simulink model "smc_controller"  (R2021a)
settings: Solver=VariableStepAuto  StartTime=0.01  StopTime=10  RelTol=1e-3
settings Model: Creator=Admin  LastModifiedBy=Admin

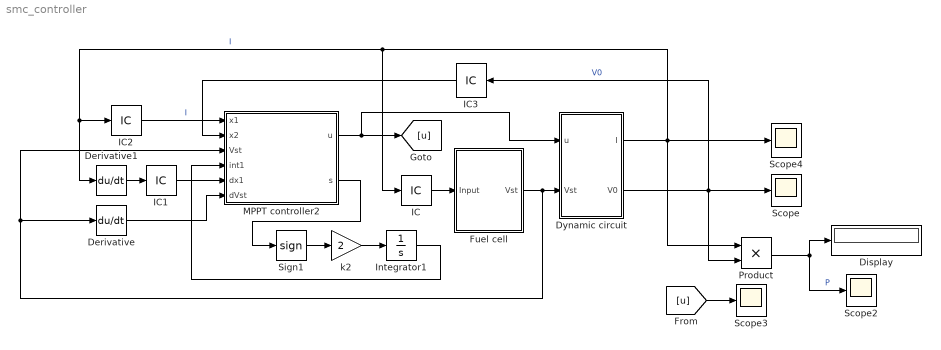
== system smc_controller ==
  Derivative : Derivative
  Derivative1 : Derivative
  Display : Display
  Dynamic circuit : Subsystem
  Fuel cell : Subsystem
  IC{,1..3} (4 alike) : InitialCondition
  Integrator1 : Integrator
  MPPT controller2 : MATLAB Function  TreatAsAtomicUnit=on
  Product : Product
  Scope{,2..4} (4 alike) : Scope
  Sign1 : Signum
  k2 : Gain  Gain=2
  wires:
  Product/1 -> Scope2/1, Display/1  "P"
  k2/1 -> Integrator1/1
  Integrator1/1 -> MPPT controller2/4(int1)
  MPPT controller2/2(s) -> Sign1/1
  Sign1/1 -> k2/1
  MPPT controller2/1(u) -> [u], Dynamic circuit/1(u)
  Dynamic circuit/1(I) -> IC/1, IC2/1, Derivative1/1, Scope4/1, Product/1  "I"
  Dynamic circuit/2(V0) -> IC3/1, Scope/1, Product/2  "V0"
  IC2/1 -> MPPT controller2/1(x1)  "I"
  Derivative1/1 -> IC1/1
  IC1/1 -> MPPT controller2/5(dx1)
  Derivative/1 -> MPPT controller2/6(dVst)
  Fuel cell/1(Vst) -> Dynamic circuit/2(Vst), MPPT controller2/3(Vst), Derivative/1
  IC/1 -> Fuel cell/1(Input)
  [u] -> Scope3/1
  IC3/1 -> MPPT controller2/2(x2)

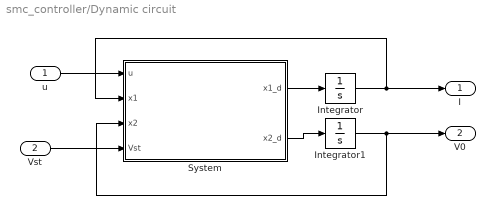
== system smc_controller/Dynamic circuit ==
  u : Inport
  Vst : Inport  Port=2
  Integrator : Integrator  InitialCondition=1
  Integrator1 : Integrator  InitialCondition=1
  System : MATLAB Function  TreatAsAtomicUnit=on
  I : Outport
  V0 : Outport  Port=2
  wires:
  System/1(x1_d) -> Integrator/1
  Integrator/1 -> I/1, System/2(x1)
  Integrator1/1 -> System/3(x2), V0/1
  System/2(x2_d) -> Integrator1/1
  u/1 -> System/1(u)
  Vst/1 -> System/4(Vst)

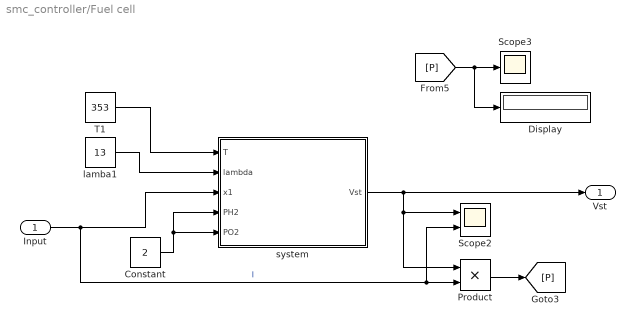
== system smc_controller/Fuel cell ==
  Input : Inport
  Constant : Constant  Value=2
  Display : Display
  Product : Product
  Scope2 : Scope  NumInputPorts=2
  Scope3 : Scope
  T1 : Constant  Value=353
  lamba1 : Constant  Value=13
  system : MATLAB Function  TreatAsAtomicUnit=on
  Vst : Outport
  wires:
  T1/1 -> system/1(T)
  Input/1 -> Product/2, Scope2/2, system/3(x1)  "I"
  system/1(Vst) -> Vst/1, Scope2/1, Product/1
  Constant/1 -> system/4(PH2), system/5(PO2)
  lamba1/1 -> system/2(lambda)
  [P] -> Display/1, Scope3/1
  Product/1 -> [P]

== matlab function smc_controller/MPPT controller2 ==
  data: u output; s output; x1 input; x2 input; Vst input; int1 input; dx1 input; dVst input
function [u,s] = MPPT_control(x1, x2, Vst, int1, dx1,dVst)
k1 = 2;
s = Vst + x1*(dVst/dx1);
u = (x2-Vst)/x2 + k1*(abs(s)).^0.5 *sign(s) + int1;

== matlab function smc_controller/Fuel cell/system ==
  data: T input; lambda input; x1 input; Vst output; PH2 input; PO2 input
function Vst = circuit(T,lambda,x1,PH2,PO2)
N = 24;
A = 232;
m1 = 0.944;
m2 = -0.00354; 
m3 = -7.8*10^-8;
m4 = 1.96*10^-4;
n = 2;
iL = 2; 
R = 83144.7; 
F = 96484600;
CO2 = PO2/((5.08*10^6)*exp(-498/T));
rm = (181.6*(1+0.03*(x1/A)+0.062*((T/303)^2)*(x1/A)^2.5))/((lambda-0.634-3*x1/A)*exp(4.18*(T-303/T))); 
tm = 175*10^-4;
Rm = rm*tm/A;
E = 1.229-8.5*(10^-4)*(T-298.15)+4.308*(10^-5)*T*(log(PH2)+log(PO2));
Vact = m1+m2*T+m3*T*log(CO2)+m4*T*log(x1);
Vohmic = x1*Rm;
Vcon = (-R*T/(n*F))*log(1-x1/(iL*A));
Vcell = E - Vact - Vohmic - Vcon;
Vst = N*Vcell;

== matlab function smc_controller/Dynamic circuit/System ==
  data: u input; x1_d output; x1 input; x2 input; x2_d output; Vst input
function [x1_d, x2_d] = circuit(u,x1,x2,Vst)
C = 7000*10^-6; 
L = 29*10^-3;
R1 = 50;
x1_d = (Vst-x2)/L + (x2/L)*u;
x2_d = x1/C - x2/(R1*C) - (x1/C)*u;
